simulink model "model"  (R2020b)
settings: Solver=VariableStepAuto  StartTime=0.0  StopTime=10  RelTol=1e-3
settings Model: Creator=SAGAR  LastModifiedBy=SAGAR

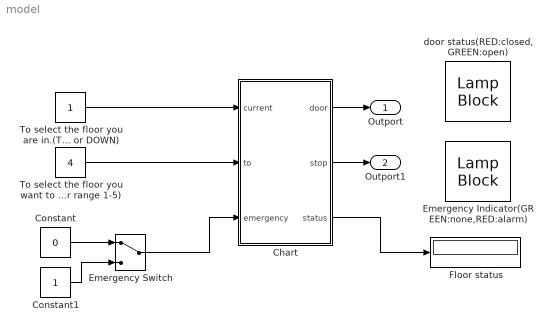
== system model ==
  Chart : Stateflow chart  TreatAsAtomicUnit=on
  Constant : Constant  Value=0
  Constant1 : Constant
  Emergency Indicator(GREEN:none,RED:alarm) : LampBlock
  Emergency Switch : ManualSwitch
  Floor status : Display
  To select the floor you are in.(To decide weather the lift will go UP or DOWN) : Constant
  To select the floor you want to go.(Floor range 1-5) : Constant  Value=4
  door status(RED:closed,GREEN:open) : LampBlock
  Outport : Outport
  Outport1 : Outport  Port=2
  wires:
  To select the floor you are in.(To decide weather the lift will go UP or DOWN)/1 -> Chart/1(current)
  Chart/1(door) -> Outport/1
  To select the floor you want to go.(Floor range 1-5)/1 -> Chart/2(to)
  Constant/1 -> Emergency Switch/1
  Constant1/1 -> Emergency Switch/2
  Emergency Switch/1 -> Chart/3(emergency)
  Chart/2(stop) -> Outport1/1
  Chart/3(status) -> Floor status/1

== stateflow chart model/Chart ==
  state LIFT
    state floor1
      entry:
      status=1;
      door=1;
      floor1=0;
      exit:
      door=0
    state control_logic
      entry:
      status;
      stop=0;
      alarm(emergency);
      floor1=0;
      restingfloor=0;
      during:
      floor1=computation(current,to);
    state floor2
      entry:
      status=2;
      door=1;
      floor1=0;
      exit:
      door=0
    state floor3
      entry:
      status=3;
      door=1;
      floor1=0;
      exit:
      door=0
    state floor4
      entry:
      status=4;
      door=1;
      floor1=0;
      exit:
      door=0
    state floor5
      entry:
      status=5;
      door=1;
      floor1=0;
      exit:
      door=0
    (default) -> control_logic
    control_logic -> floor1 [order 1] : [floor1==1]
    floor1 -> control_logic : after(9.4,sec)[floor1==0]
    control_logic -> floor2 [order 2] : [floor1==2]
    floor2 -> control_logic : after(9.4,sec)[floor1==0]
    control_logic -> floor3 [order 3] : [floor1==3]
    floor3 -> control_logic : after(9.4,sec)[floor1==0]
    control_logic -> floor4 [order 4] : [floor1==4]
    floor4 -> control_logic : after(9.4,sec)[floor1==0]
    control_logic -> floor5 [order 5] : [floor1==5]
    floor5 -> control_logic : after(9.4,sec)[floor1==0]
  state floorx=computation(current1,to1) [function]
    (default) -> (junction 16) : % current floor and to floor
    (junction 16) -> (junction 17) [order 1] : [current1>to1]
    (junction 17) -> (junction 19) : {floorx=current1-to1;
        | current1=current1-floorx;
        | floorx=current1;;}
    (junction 16) -> (junction 18) [order 2] : {floorx=to1-current1;
        | current1=current1+floorx;
        | floorx=current1;}
    (junction 19) -> (junction 18)
    (junction 18) -> (junction 20)
  state alarm(emergency1) [function]
    (default) -> (junction 78) : % alarm
    (junction 78) -> (junction 79) [order 1] : [emergency1==1]
    (junction 78) -> (junction 80) [order 2]
    (junction 79) -> (junction 81) : {door=1;
        | stop=1;}
    (junction 81) -> (junction 80)
    (junction 80) -> (junction 82)
  data: current1 function_input; to1 function_input; floorx function_output; emergency1 function_input; current input; to input; floor1 local; restingfloor local; door output; stop output; emergency input; status output
